simulink model "Laboratory_3_2_block"  (R2023b)
settings: Solver=VariableStepAuto  StartTime=0.0  StopTime=10.0  RelTol=1e-3
values from neighbouring files (symbols this model uses):
  G1_den = [1 0 0]    [Laboratory_3_1.m]    (also in Laboratory_3_2.m)
  G1_num = [1]    [Laboratory_3_1.m]    (also in Laboratory_3_2.m)
  G2_den = [1 1]    [Laboratory_3_1.m]    (also in Laboratory_3_2.m)
  G2_num = [1]    [Laboratory_3_1.m]    (also in Laboratory_3_2.m)
  G3_den = [1 0]    [Laboratory_3_1.m]    (also in Laboratory_3_2.m)
  G3_num = [1]    [Laboratory_3_1.m]    (also in Laboratory_3_2.m)
  G4_den = [1 -1 0 0 1 -2 1]    [Laboratory_3_1.m]    (also in Laboratory_3_2.m = [2 0])
  G4_num = [1 0 -4 0]    [Laboratory_3_1.m]    (also in Laboratory_3_2.m = [1])
  G5_den = [8 0 -32 -4 32 -8 -20 -8 -12 4 8 0 0 0 0 0 0 0]    [Laboratory_3_2.m]
  G5_num = [4 -4 -12 4 8 0 0 0 0 0 0 0 0]    [Laboratory_3_2.m]
  H1_den = [1 0]    [Laboratory_3_1.m]    (also in Laboratory_3_2.m)
  H1_num = [1]    [Laboratory_3_1.m]    (also in Laboratory_3_2.m)
  H2_den = [1 -1]    [Laboratory_3_1.m]    (also in Laboratory_3_2.m)
  H2_num = [1]    [Laboratory_3_1.m]    (also in Laboratory_3_2.m)
  H3_den = [1 -2]    [Laboratory_3_1.m]    (also in Laboratory_3_2.m)
  H3_num = [1]    [Laboratory_3_1.m]    (also in Laboratory_3_2.m)
settings Model: Creator=USER  LastModifiedBy=trist

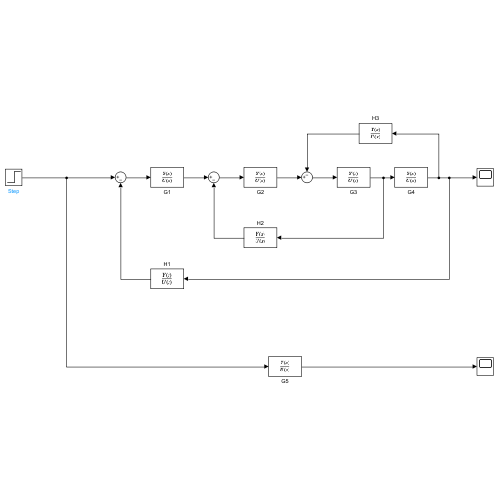
[thumbnail: Simulink's stored preview of the top-level diagram]
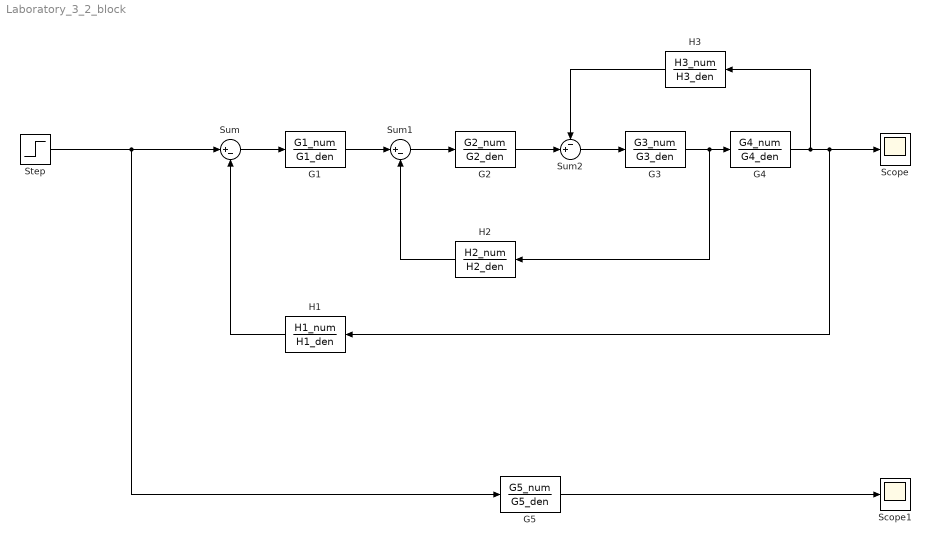
== system Laboratory_3_2_block ==
  G1 : TransferFcn  Numerator=G1_num  Denominator=G1_den
  G2 : TransferFcn  Numerator=G2_num  Denominator=G2_den
  G3 : TransferFcn  Numerator=G3_num  Denominator=G3_den
  G4 : TransferFcn  Numerator=G4_num  Denominator=G4_den
  G5 : TransferFcn  Numerator=G5_num  Denominator=G5_den
  H1 : TransferFcn  Numerator=H1_num  Denominator=H1_den
  H2 : TransferFcn  Numerator=H2_num  Denominator=H2_den
  H3 : TransferFcn  Numerator=H3_num  Denominator=H3_den
  Scope : Scope
  Scope1 : Scope
  Step : Step  SampleTime=0
  Sum : Sum  Inputs=|+-
  Sum1 : Sum  Inputs=|+-
  Sum2 : Sum  Inputs=-+|
  wires:
  Sum/1 -> G1/1
  G1/1 -> Sum1/1
  Sum1/1 -> G2/1
  H1/1 -> Sum/2
  H2/1 -> Sum1/2
  Sum2/1 -> G3/1
  G2/1 -> Sum2/2
  G3/1 -> H2/1, G4/1
  G4/1 -> H3/1, H1/1, Scope/1
  H3/1 -> Sum2/1
  Step/1 -> G5/1, Sum/1
  G5/1 -> Scope1/1
